simulink model "Ilabexample_water_clock"  (R2016a)
settings: Solver=VariableStepAuto  StartTime=0.0  StopTime=86400  RelTol=1e-3
undefined symbols (not defined in the file or in its folder): A2, A3, Hr, K1, K2
settings Model: Creator=tomevetts  LastModifiedBy=tomevetts

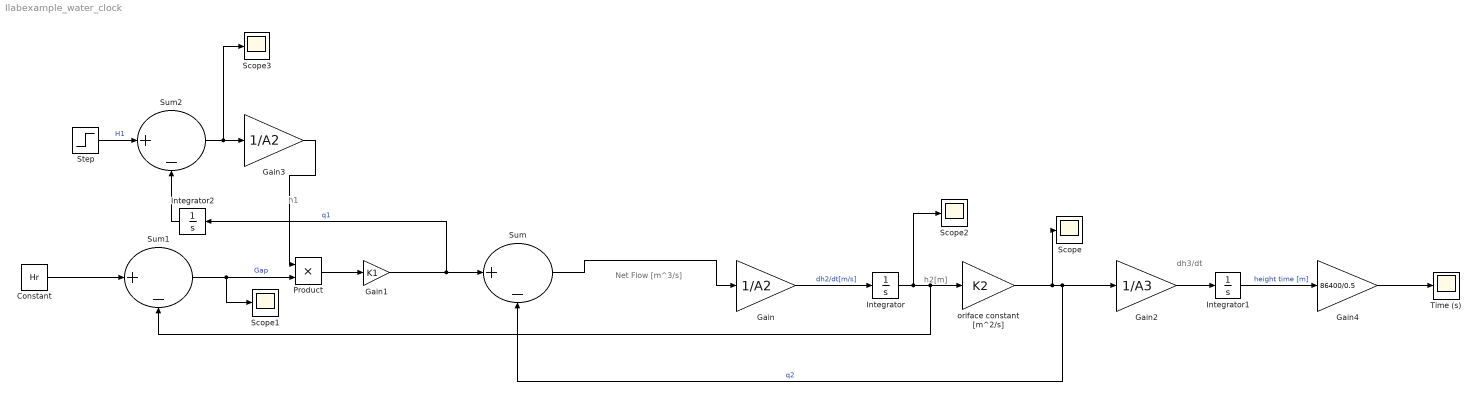
== system Ilabexample_water_clock ==
  note: h1
  note: dh3/dt
  note: h2[m]
  note: Net Flow [m^3/s]
  Constant : Constant  Value=Hr
  Gain : Gain  Gain=1/A2
  Gain1 : Gain  Gain=K1
  Gain2 : Gain  Gain=1/A3
  Gain3 : Gain  Gain=1/A2
  Gain4 : Gain  Gain=86400/0.5
  Integrator : Integrator
  Integrator1 : Integrator
  Integrator2 : Integrator
  Product : Product
  Scope{,1..3} (4 alike) : Scope
  Step : Step  Time=0  After=0.01  SampleTime=0
  Sum : Sum  Inputs=|+-
  Sum1 : Sum  Inputs=|+-
  Sum2 : Sum  Inputs=|+-
  Time (s) : Scope
  oriface constant [m^2/s] : Gain  Gain=K2
  wires:
  oriface constant [m^2/s]/1 -> Scope/1, Gain2/1, Sum/2  "q2"
  Gain1/1 -> Integrator2/1, Sum/1  "q1"
  Sum/1 -> Gain/1
  Gain/1 -> Integrator/1  "dh2/dt[m/s]"
  Product/1 -> Gain1/1
  Sum1/1 -> Scope1/1, Product/2  "Gap"
  Integrator/1 -> Scope2/1, Sum1/2, oriface constant [m^2/s]/1
  Constant/1 -> Sum1/1
  Gain2/1 -> Integrator1/1
  Integrator1/1 -> Gain4/1  "height time [m]"
  Step/1 -> Sum2/1  "H1"
  Sum2/1 -> Scope3/1, Gain3/1
  Gain3/1 -> Product/1
  Integrator2/1 -> Sum2/2
  Gain4/1 -> Time (s)/1
